simulink model "exp9"  (R2025b)
settings: Solver=VariableStepAuto  StartTime=0.0  StopTime=10.0  RelTol=1e-3
libraries: simulink_extras x4
settings Model: Creator=shanm  LastModifiedBy=SUBHASH

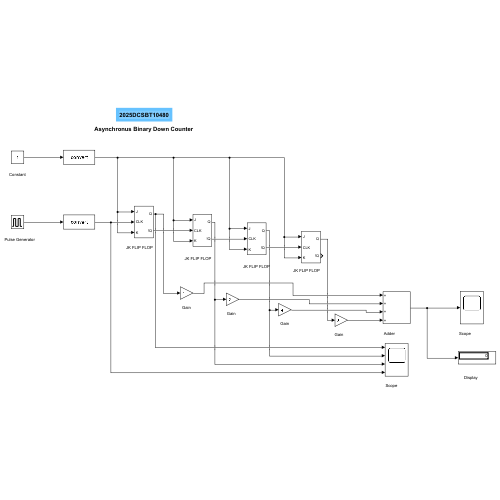
[thumbnail: Simulink's stored preview of the top-level diagram]
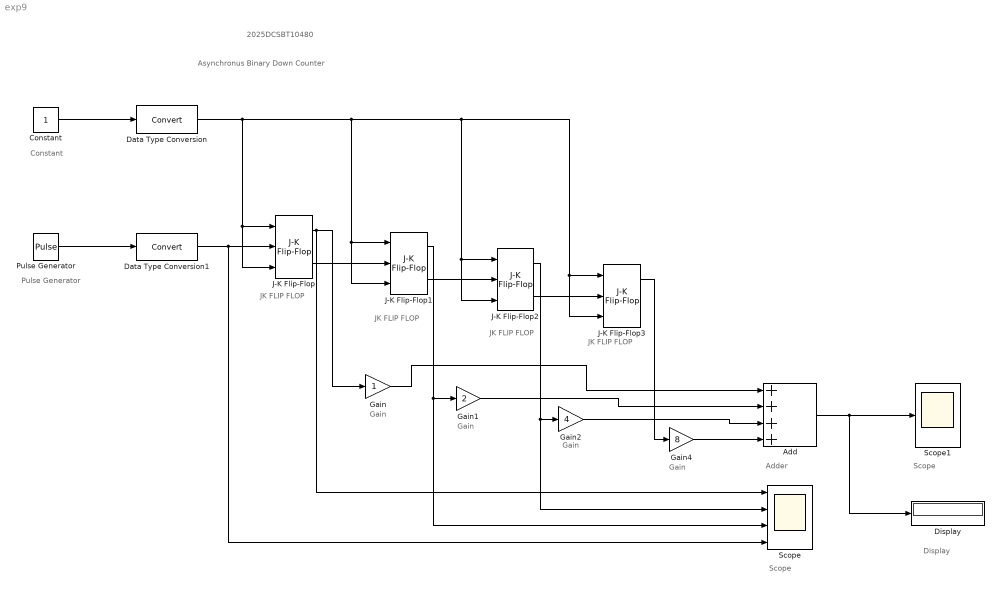
== system exp9 ==
  note: JK FLIP FLOP
  note: Constant
  note: Pulse Generator
  note: Adder
  note: Scope
  note: Scope
  note: Display
  note: 2025DCSBT10480
  note: Asynchronus Binary Down Counter
  note: Gain
  note: Gain
  note: Gain
  note: Gain
  note: JK FLIP FLOP
  note: JK FLIP FLOP
  note: JK FLIP FLOP
  Add : Sum  Inputs=++++
  Constant : Constant
  Data Type Conversion : DataTypeConversion  SaturateOnIntegerOverflow=off  RndMeth=Floor
  Data Type Conversion1 : DataTypeConversion  SaturateOnIntegerOverflow=off  RndMeth=Floor
  Display : Display
  Gain : Gain
  Gain1 : Gain  Gain=2
  Gain2 : Gain  Gain=4
  Gain4 : Gain  Gain=8
  J-K Flip-Flop{,1..3} (4 alike) : simulink_extras/Flip Flops/J-K Flip-Flop  initial_condition=0
  Pulse Generator : DiscretePulseGenerator  PulseType=Time based  Period=1  PulseWidth=50
  Scope : Scope  NumInputPorts=4
      settings: ActiveDisplayYMinimum=-1  ActiveDisplayYMaximum=1
  Scope1 : Scope
      settings: ActiveDisplayYMinimum=2.3034831137686975  ActiveDisplayYMaximum=8.62764207605834
  wires:
  Pulse Generator/1 -> Data Type Conversion1/1
  Data Type Conversion1/1 -> Scope/4, J-K Flip-Flop/2
  Constant/1 -> Data Type Conversion/1
  Data Type Conversion/1 -> J-K Flip-Flop/3, J-K Flip-Flop/1, J-K Flip-Flop1/3, J-K Flip-Flop1/1, J-K Flip-Flop2/3, J-K Flip-Flop2/1, J-K Flip-Flop3/3, J-K Flip-Flop3/1
  J-K Flip-Flop/2 -> J-K Flip-Flop1/2
  J-K Flip-Flop1/2 -> J-K Flip-Flop2/2
  J-K Flip-Flop2/2 -> J-K Flip-Flop3/2
  J-K Flip-Flop2/1 -> Gain2/1, Scope/2
  J-K Flip-Flop3/1 -> Gain4/1
  Gain4/1 -> Add/4
  J-K Flip-Flop1/1 -> Gain1/1, Scope/3
  Gain/1 -> Add/1
  J-K Flip-Flop/1 -> Gain/1, Scope/1
  Add/1 -> Display/1, Scope1/1
  Gain1/1 -> Add/2
  Gain2/1 -> Add/3
